simulink model "PubIfDecisionVSM_ISL"  (R2020b)
settings: Solver=FixedStepAuto  StartTime=0.0  StopTime=Inf  RelTol=1e-3
PostLoadFcn:
  | if any(exist('dsrtsu_mdlpostloadfcn', 'file') ~= 0), dsrtsu_mdlpostloadfcn('Execute', bdroot); end
InitFcn:
  | , if any(exist('dsmpb_private', 'file') ~= 0), dsmpb_private('dsmpb_mdlclblib', 'Init', bdroot); end,
PreSaveFcn:
  | , if any(exist('dsmpb_private', 'file') ~= 0), dsmpb_private('dsmpb_mdlclblib', 'PreSave', bdroot); end,
CloseFcn:
  | , if any(exist('dsmpb_private', 'file') ~= 0), dsmpb_private('dsmpb_mdlclblib', 'Close', bdroot); end,
settings Model: DataDictionary=HWA_DDs.sldd  RTICANMMDATA=struct('GeneralSetupData',struct('modelroot','D:\ADAS_Store\Adas\VSM\ISL','generalsettings',struct('filesettings',struct('destfolder',struct('Name','RTICANMM_FILES','Check',1),'buildfolder',struct('Name','.','Check',1),'AbsDestfolder',struct('Name','D:\ADAS_Store\Adas\VSM\ISL\RTICANMM_FILES'),'AbsBuildfolder',struct('Name','D:\ADAS_Store\Adas\VSM\ISL'))),'options',struct('addpaths',1,'rmpaths',1,'addtrcexclusion',false,'cannavigator',struct('checkmonitoring',0),'show_usrtrc',0,'use_usrtrc',0),'advanced',struct('options',ones(1,100)),'MPSetup',{{}},'RTI',struct('Type','DSRT','Ver','4.2','Date','02-Nov-2019'),'modelname','PubIfDecisionVSM_ISL','block','PubIfDecisionVSM_ISL'))  DSRTSU_INTERNAL_RTIFPGA=150  Creator=GW00180895  LastModifiedBy=GW00166368
settings OptimizationCC: BlockReduction=off  ConditionallyExecuteInputs=off  OptimizeBlockIOStorage=off  BufferReuse=off  GlobalBufferReuse=off  ExpressionFolding=off  LocalBlockOutputs=off  OptimizeDataStoreBuffers=off  BusAssignmentInplaceUpdate=off
settings DebuggingCC: TasksWithSamePriorityMsg=none
settings HardwareCC: ProdBitPerPointer=32  ProdBitPerSizeT=32  ProdBitPerPtrDiffT=32  ProdLargestAtomicInteger=Integer  ProdWordSize=32  ProdHWDeviceType=Custom Processor->Custom
settings ModelReferenceCC: UpdateModelReferenceTargets=IfOutOfDate  EnableParallelModelReferenceBuilds=on  ModelReferenceNumInstancesAllowed=Single
settings SFSimCC: MATLABDynamicMemAlloc=off
settings RTWCC: Description=dSPACE Run-Time Target (for VEOS on Windows and ConfigurationDesk)  SystemTargetFile=dsrt.tlc  GenCodeOnly=on  MakeCommand=make_dsrt  TemplateMakefile=dsrt_default_tmf  RTWVerbose=off
settings CodeAppCC: MaxIdLength=128
settings STFCustomTargetCC: TargetLangStandard=C99 (ISO)  ParMdlRefBuildCompliant=on  ConcurrentExecutionCompliant=off  CPPClassGenCompliant=off  GRTInterface=off  SystemTargetFile=dsrt.tlc
settings GRTTargetCC: CompOptLevelCompliant=off  ConcurrentExecutionCompliant=off  CombineOutputUpdateFcns=off  MatFileLogging=off  CPPClassGenCompliant=off  UseToolchainInfoCompliant=off

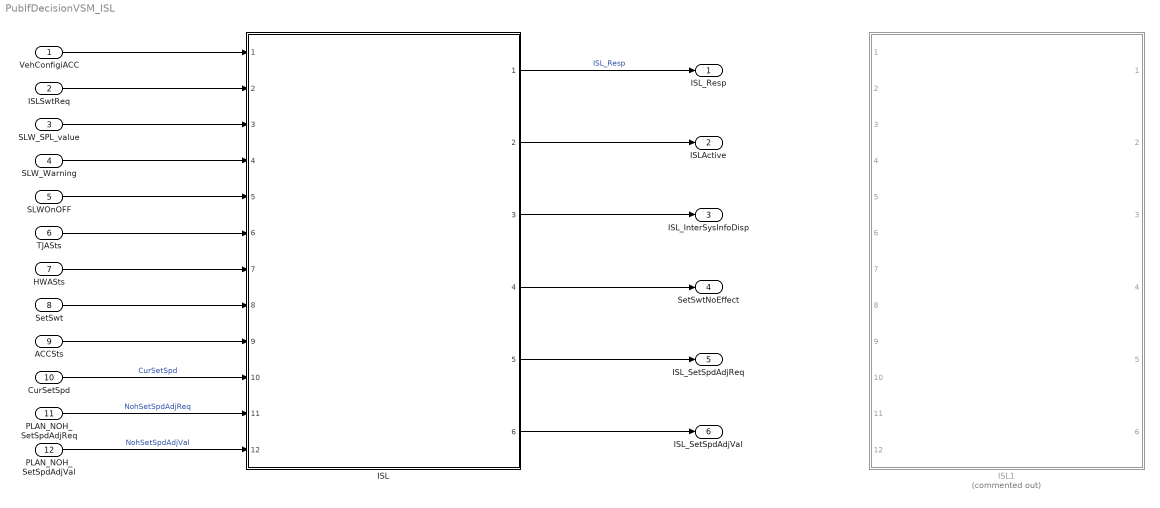
== system PubIfDecisionVSM_ISL ==
  VehConfigiACC : Inport  OutDataTypeStr=uint8
  ISLSwtReq : Inport  Port=2  OutDataTypeStr=boolean
  SLW_SPL_value : Inport  Port=3  OutDataTypeStr=uint8
  SLW_Warning : Inport  Port=4  OutDataTypeStr=boolean
  SLWOnOFF : Inport  Port=5  OutDataTypeStr=boolean
  TJASts : Inport  Port=6  OutDataTypeStr=Enum: TJA_STATE
  HWASts : Inport  Port=7  OutDataTypeStr=Enum: HWA_STATE
  SetSwt : Inport  Port=8  OutDataTypeStr=boolean
  ACCSts : Inport  Port=9  OutDataTypeStr=Enum: ACC_STATE
  CurSetSpd : Inport  Port=10  OutDataTypeStr=single
  PLAN_NOH_SetSpdAdjReq : Inport  Port=11  OutDataTypeStr=boolean
  PLAN_NOH_SetSpdAdjVal : Inport  Port=12  OutDataTypeStr=uint8
  ISL : Subsystem  ReferencedSubsystem=SubSystem_VSM_ISL
  ISL1 : Subsystem  Commented=on  ReferencedSubsystem=SubSystem_VSM_ISL
  ISL_Resp : Outport  OutDataTypeStr=boolean
  ISLActive : Outport  Port=2  OutDataTypeStr=boolean
  ISL_InterSysInfoDisp : Outport  Port=3  OutDataTypeStr=uint8
  SetSwtNoEffect : Outport  Port=4  OutDataTypeStr=boolean
  ISL_SetSpdAdjReq : Outport  Port=5  OutDataTypeStr=boolean
  ISL_SetSpdAdjVal : Outport  Port=6  OutDataTypeStr=uint8
  wires:
  ISLSwtReq/1 -> ISL/2
  SLW_SPL_value/1 -> ISL/3
  HWASts/1 -> ISL/7
  SetSwt/1 -> ISL/8
  ACCSts/1 -> ISL/9
  VehConfigiACC/1 -> ISL/1
  SLW_Warning/1 -> ISL/4
  CurSetSpd/1 -> ISL/10  "CurSetSpd"
  TJASts/1 -> ISL/6
  SLWOnOFF/1 -> ISL/5
  ISL/2 -> ISLActive/1
  ISL/1 -> ISL_Resp/1  "ISL_Resp"
  ISL/4 -> SetSwtNoEffect/1
  ISL/3 -> ISL_InterSysInfoDisp/1
  ISL/5 -> ISL_SetSpdAdjReq/1
  ISL/6 -> ISL_SetSpdAdjVal/1
  PLAN_NOH_SetSpdAdjReq/1 -> ISL/11  "NohSetSpdAdjReq"
  PLAN_NOH_SetSpdAdjVal/1 -> ISL/12  "NohSetSpdAdjVal"
